simulink model "diffusion"  (R2021b)
settings: Solver=ode4  StartTime=0.0  StopTime=100  FixedStep=1E-3  RelTol=1e-3
values from neighbouring files (symbols this model uses):
  A = [0 1 1 1 1 1 1 1 1 1 1 1 ... (16384 elements, 128x128)]    [centered_distribution.mat]    (also in discussionSami.mat = [0 0 0 0 1 0 1 1 0 1 1 0 ... (16384 elements, 128x128)]; newResultsMoreRobots_1.mat; scrpt_collective_learning_dynamics_v4.m = A.*(~eye(size(A))); test50gammas_eta_n0.1.mat)
  L = D - A    [scrpt_collective_learning_dynamics_v4.m]
  N = 3    [scrpt_collective_learning_dynamics_v4.m]    (also in scrpt_math_framework_v4.m = 1:1:1000)
settings Model: Creator=diaz  LastModifiedBy=diaz

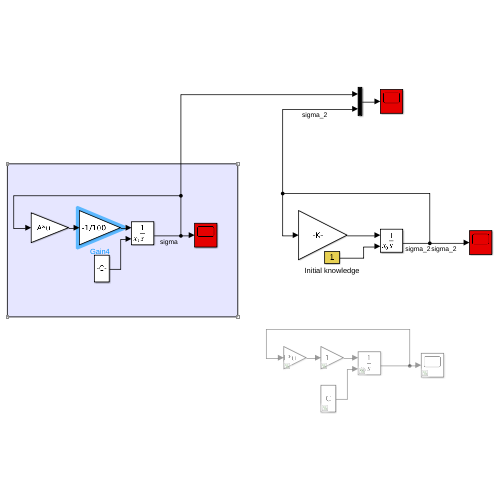
[thumbnail: Simulink's stored preview of the top-level diagram]
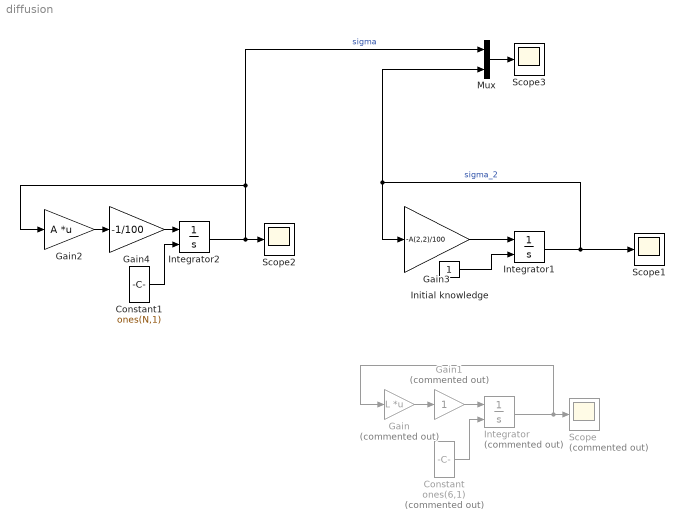
== system diffusion ==
  Constant : Constant  Commented=on  Value=ones(6,1)
  Constant1 : Constant  Value=ones(N,1)
  Gain : Gain  Commented=on  Gain=L  Multiplication=Matrix(K*u)
  Gain1 : Gain  Commented=on
  Gain2 : Gain  Gain=A  Multiplication=Matrix(K*u)
  Gain3 : Gain  Gain=-A(2,2)/100
  Gain4 : Gain  Gain=-1/100
  Initial knowledge : Constant
  Integrator : Integrator  Commented=on  InitialConditionSource=external  InitialCondition=1
  Integrator1 : Integrator  InitialConditionSource=external  InitialCondition=1
  Integrator2 : Integrator  InitialConditionSource=external  InitialCondition=1
  Mux : Mux  Inputs=2
  Scope : Scope  Commented=on
  Scope1 : Scope
  Scope2 : Scope
  Scope3 : Scope
  wires:
  Gain/1 -> Gain1/1
  Constant/1 -> Integrator/2
  Integrator/1 -> Gain/1, Scope/1
  Gain1/1 -> Integrator/1
  Gain3/1 -> Integrator1/1
  Integrator1/1 -> Scope1/1, Mux/2, Gain3/1  "sigma_2"
  Initial knowledge/1 -> Integrator1/2
  Integrator2/1 -> Scope2/1, Mux/1, Gain2/1  "sigma"
  Gain4/1 -> Integrator2/1
  Gain2/1 -> Gain4/1
  Constant1/1 -> Integrator2/2
  Mux/1 -> Scope3/1
